simulink model "mmc_hb_switching"  (R2026a)
settings: Solver=ode3  StopTime=Tstop  FixedStep=Ts_elec
undefined symbols (not defined in the file): topology_id, Vdc, Vphase_cmd
libraries: fl_lib x23, nesl_utility x23, ee_lib x11
settings Model: Creator=zheng  LastModifiedBy=zheng

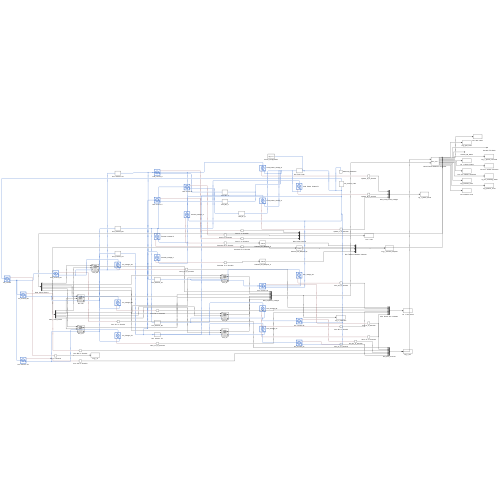
[thumbnail: Simulink's stored preview of the top-level diagram]
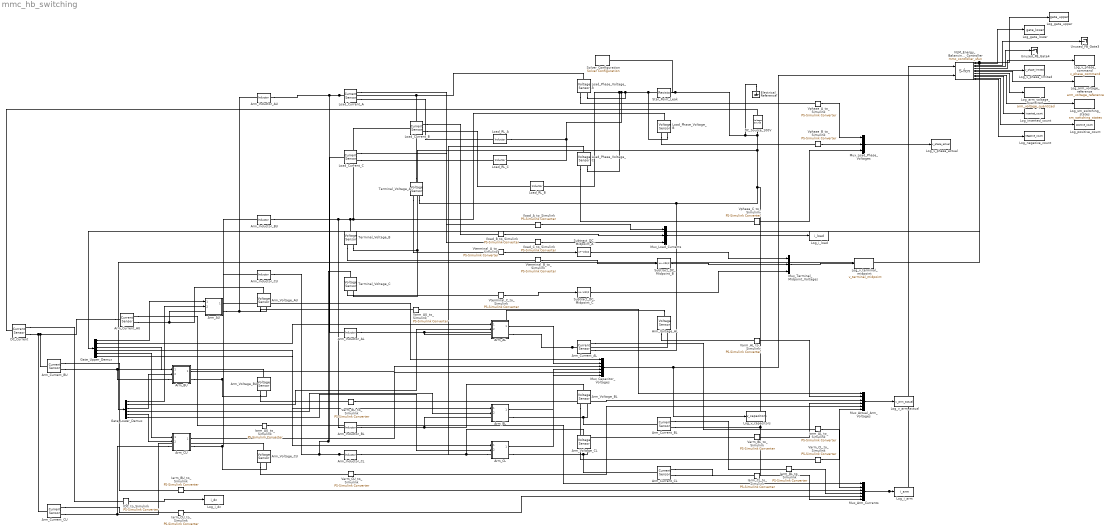
== system mmc_hb_switching ==
  Arm_AL : Subsystem  ReferencedSubsystem=mmc_hb_arm
  Arm_AU : Subsystem  ReferencedSubsystem=mmc_hb_arm
  Arm_BL : Subsystem  ReferencedSubsystem=mmc_hb_arm
  Arm_BU : Subsystem  ReferencedSubsystem=mmc_hb_arm
  Arm_CL : Subsystem  ReferencedSubsystem=mmc_hb_arm
  Arm_CU : Subsystem  ReferencedSubsystem=mmc_hb_arm
  Arm_Current_AL : fl_lib/Electrical/Electrical Sensors/Current Sensor
  Arm_Current_AU : fl_lib/Electrical/Electrical Sensors/Current Sensor
  Arm_Current_BL : fl_lib/Electrical/Electrical Sensors/Current Sensor
  Arm_Current_BU : fl_lib/Electrical/Electrical Sensors/Current Sensor
  Arm_Current_CL : fl_lib/Electrical/Electrical Sensors/Current Sensor
  Arm_Current_CU : fl_lib/Electrical/Electrical Sensors/Current Sensor
  Arm_Inductor_AL : ee_lib/Passive/Inductor  l=Larm H  enable_L_tol=ee.enum.toleranceApplication.none  L_tol=20  tol_distribution=ee.enum.toleranceDistribution.uniform  nSigma=4  r=Rarm Ohm  g=1e-9 1/Ohm  enable_operating_limits=ee.enum.enable.no  operating_limit_action=ee.enum.passive.reportOpLim.warn  max_working_current=1 A  power_rating=1 W  i_L_specify=off  i_L_priority=High  i_L=0 A  i_L_nominal_specify=off  i_L_nominal_value=1  i_L_nominal_unit=A
  Arm_Inductor_AU : ee_lib/Passive/Inductor  l=Larm H  enable_L_tol=ee.enum.toleranceApplication.none  L_tol=20  tol_distribution=ee.enum.toleranceDistribution.uniform  nSigma=4  r=Rarm Ohm  g=1e-9 1/Ohm  enable_operating_limits=ee.enum.enable.no  operating_limit_action=ee.enum.passive.reportOpLim.warn  max_working_current=1 A  power_rating=1 W  i_L_specify=off  i_L_priority=High  i_L=0 A  i_L_nominal_specify=off  i_L_nominal_value=1  i_L_nominal_unit=A
  Arm_Inductor_BL : ee_lib/Passive/Inductor  l=Larm H  enable_L_tol=ee.enum.toleranceApplication.none  L_tol=20  tol_distribution=ee.enum.toleranceDistribution.uniform  nSigma=4  r=Rarm Ohm  g=1e-9 1/Ohm  enable_operating_limits=ee.enum.enable.no  operating_limit_action=ee.enum.passive.reportOpLim.warn  max_working_current=1 A  power_rating=1 W  i_L_specify=off  i_L_priority=High  i_L=0 A  i_L_nominal_specify=off  i_L_nominal_value=1  i_L_nominal_unit=A
  Arm_Inductor_BU : ee_lib/Passive/Inductor  l=Larm H  enable_L_tol=ee.enum.toleranceApplication.none  L_tol=20  tol_distribution=ee.enum.toleranceDistribution.uniform  nSigma=4  r=Rarm Ohm  g=1e-9 1/Ohm  enable_operating_limits=ee.enum.enable.no  operating_limit_action=ee.enum.passive.reportOpLim.warn  max_working_current=1 A  power_rating=1 W  i_L_specify=off  i_L_priority=High  i_L=0 A  i_L_nominal_specify=off  i_L_nominal_value=1  i_L_nominal_unit=A
  Arm_Inductor_CL : ee_lib/Passive/Inductor  l=Larm H  enable_L_tol=ee.enum.toleranceApplication.none  L_tol=20  tol_distribution=ee.enum.toleranceDistribution.uniform  nSigma=4  r=Rarm Ohm  g=1e-9 1/Ohm  enable_operating_limits=ee.enum.enable.no  operating_limit_action=ee.enum.passive.reportOpLim.warn  max_working_current=1 A  power_rating=1 W  i_L_specify=off  i_L_priority=High  i_L=0 A  i_L_nominal_specify=off  i_L_nominal_value=1  i_L_nominal_unit=A
  Arm_Inductor_CU : ee_lib/Passive/Inductor  l=Larm H  enable_L_tol=ee.enum.toleranceApplication.none  L_tol=20  tol_distribution=ee.enum.toleranceDistribution.uniform  nSigma=4  r=Rarm Ohm  g=1e-9 1/Ohm  enable_operating_limits=ee.enum.enable.no  operating_limit_action=ee.enum.passive.reportOpLim.warn  max_working_current=1 A  power_rating=1 W  i_L_specify=off  i_L_priority=High  i_L=0 A  i_L_nominal_specify=off  i_L_nominal_value=1  i_L_nominal_unit=A
  Arm_Voltage_AL : fl_lib/Electrical/Electrical Sensors/Voltage Sensor
  Arm_Voltage_AU : fl_lib/Electrical/Electrical Sensors/Voltage Sensor
  Arm_Voltage_BL : fl_lib/Electrical/Electrical Sensors/Voltage Sensor
  Arm_Voltage_BU : fl_lib/Electrical/Electrical Sensors/Voltage Sensor
  Arm_Voltage_CL : fl_lib/Electrical/Electrical Sensors/Voltage Sensor
  Arm_Voltage_CU : fl_lib/Electrical/Electrical Sensors/Voltage Sensor
  DC_Current : fl_lib/Electrical/Electrical Sensors/Current Sensor
  DC_Source_100V : ee_lib/Sources/Voltage Source  dc_voltage=Vdc V  ac_voltage=0 V  ac_shift=0 rad  ac_frequency=60 Hz  noise_mode=ee.enum.sources.noise.Disabled  PSD=0 V^2/Hz  sample_time=1e-3 s  repeatability=ee.enum.sources.repeatability.NotRepeatable  user_seed=0  auto_seed=545404223  i_specify=off  i_priority=None  i=0 A  i_nominal_specify=off  i_nominal_value=1  i_nominal_unit=A  v_specify=off  v_priority=None  v=Vdc V  v_nominal_specify=off  v_nominal_value=1  v_nominal_unit=V
  Electrical_Reference : fl_lib/Electrical/Electrical Elements/Electrical Reference
  Gate_Lower_Demux : Demux  Outputs=[10 10 10 10 10 10]
  Gate_Upper_Demux : Demux  Outputs=[10 10 10 10 10 10]
  IDC_to_Simulink : nesl_utility/PS-Simulink Converter  PhysicalDomain=network_engine_domain  SubClassName=ps_output  LeftPortType=input  RightPortType=output  PseudoPeriodic=off  Frequencies=[]  VectorFormat=inherit  Unit=A  AffineConversion=off
  Iarm_AL_to_Simulink : nesl_utility/PS-Simulink Converter  PhysicalDomain=network_engine_domain  SubClassName=ps_output  LeftPortType=input  RightPortType=output  PseudoPeriodic=off  Frequencies=[]  VectorFormat=inherit  Unit=A  AffineConversion=off
  Iarm_AU_to_Simulink : nesl_utility/PS-Simulink Converter  PhysicalDomain=network_engine_domain  SubClassName=ps_output  LeftPortType=input  RightPortType=output  PseudoPeriodic=off  Frequencies=[]  VectorFormat=inherit  Unit=A  AffineConversion=off
  Iarm_BL_to_Simulink : nesl_utility/PS-Simulink Converter  PhysicalDomain=network_engine_domain  SubClassName=ps_output  LeftPortType=input  RightPortType=output  PseudoPeriodic=off  Frequencies=[]  VectorFormat=inherit  Unit=A  AffineConversion=off
  Iarm_BU_to_Simulink : nesl_utility/PS-Simulink Converter  PhysicalDomain=network_engine_domain  SubClassName=ps_output  LeftPortType=input  RightPortType=output  PseudoPeriodic=off  Frequencies=[]  VectorFormat=inherit  Unit=A  AffineConversion=off
  Iarm_CL_to_Simulink : nesl_utility/PS-Simulink Converter  PhysicalDomain=network_engine_domain  SubClassName=ps_output  LeftPortType=input  RightPortType=output  PseudoPeriodic=off  Frequencies=[]  VectorFormat=inherit  Unit=A  AffineConversion=off
  Iarm_CU_to_Simulink : nesl_utility/PS-Simulink Converter  PhysicalDomain=network_engine_domain  SubClassName=ps_output  LeftPortType=input  RightPortType=output  PseudoPeriodic=off  Frequencies=[]  VectorFormat=inherit  Unit=A  AffineConversion=off
  Iload_A_to_Simulink : nesl_utility/PS-Simulink Converter  PhysicalDomain=network_engine_domain  SubClassName=ps_output  LeftPortType=input  RightPortType=output  PseudoPeriodic=off  Frequencies=[]  VectorFormat=inherit  Unit=A  AffineConversion=off
  Iload_B_to_Simulink : nesl_utility/PS-Simulink Converter  PhysicalDomain=network_engine_domain  SubClassName=ps_output  LeftPortType=input  RightPortType=output  PseudoPeriodic=off  Frequencies=[]  VectorFormat=inherit  Unit=A  AffineConversion=off
  Iload_C_to_Simulink : nesl_utility/PS-Simulink Converter  PhysicalDomain=network_engine_domain  SubClassName=ps_output  LeftPortType=input  RightPortType=output  PseudoPeriodic=off  Frequencies=[]  VectorFormat=inherit  Unit=A  AffineConversion=off
  Load_Current_A : fl_lib/Electrical/Electrical Sensors/Current Sensor
  Load_Current_B : fl_lib/Electrical/Electrical Sensors/Current Sensor
  Load_Current_C : fl_lib/Electrical/Electrical Sensors/Current Sensor
  Load_Phase_Voltage_A : fl_lib/Electrical/Electrical Sensors/Voltage Sensor
  Load_Phase_Voltage_B : fl_lib/Electrical/Electrical Sensors/Voltage Sensor
  Load_Phase_Voltage_C : fl_lib/Electrical/Electrical Sensors/Voltage Sensor
  Load_RL_A : ee_lib/Passive/Inductor  l=Lload H  enable_L_tol=ee.enum.toleranceApplication.none  L_tol=20  tol_distribution=ee.enum.toleranceDistribution.uniform  nSigma=4  r=Rload Ohm  g=1e-9 1/Ohm  enable_operating_limits=ee.enum.enable.no  operating_limit_action=ee.enum.passive.reportOpLim.warn  max_working_current=1 A  power_rating=1 W  i_L_specify=off  i_L_priority=High  i_L=0 A  i_L_nominal_specify=off  i_L_nominal_value=1  i_L_nominal_unit=A
  Load_RL_B : ee_lib/Passive/Inductor  l=Lload H  enable_L_tol=ee.enum.toleranceApplication.none  L_tol=20  tol_distribution=ee.enum.toleranceDistribution.uniform  nSigma=4  r=Rload Ohm  g=1e-9 1/Ohm  enable_operating_limits=ee.enum.enable.no  operating_limit_action=ee.enum.passive.reportOpLim.warn  max_working_current=1 A  power_rating=1 W  i_L_specify=off  i_L_priority=High  i_L=0 A  i_L_nominal_specify=off  i_L_nominal_value=1  i_L_nominal_unit=A
  Load_RL_C : ee_lib/Passive/Inductor  l=Lload H  enable_L_tol=ee.enum.toleranceApplication.none  L_tol=20  tol_distribution=ee.enum.toleranceDistribution.uniform  nSigma=4  r=Rload Ohm  g=1e-9 1/Ohm  enable_operating_limits=ee.enum.enable.no  operating_limit_action=ee.enum.passive.reportOpLim.warn  max_working_current=1 A  power_rating=1 W  i_L_specify=off  i_L_priority=High  i_L=0 A  i_L_nominal_specify=off  i_L_nominal_value=1  i_L_nominal_unit=A
  Log_arm_voltage_quantized : ToWorkspace  VariableName=arm_voltage_quantized  SaveFormat=Timeseries  SampleTime=-1
  Log_arm_voltage_reference : ToWorkspace  VariableName=arm_voltage_reference  SaveFormat=Timeseries  SampleTime=-1
  Log_gate_lower : ToWorkspace  VariableName=gate_lower  SaveFormat=Timeseries  SampleTime=-1
  Log_gate_upper : ToWorkspace  VariableName=gate_upper  SaveFormat=Timeseries  SampleTime=-1
  Log_i_arm : ToWorkspace  VariableName=i_arm  SaveFormat=Timeseries  SampleTime=-1
  Log_i_dc : ToWorkspace  VariableName=i_dc  SaveFormat=Timeseries  SampleTime=-1
  Log_i_load : ToWorkspace  VariableName=i_load  SaveFormat=Timeseries  SampleTime=-1
  Log_inserted_count : ToWorkspace  VariableName=inserted_count  SaveFormat=Timeseries  SampleTime=-1
  Log_negative_count : ToWorkspace  VariableName=negative_count  SaveFormat=Timeseries  SampleTime=-1
  Log_positive_count : ToWorkspace  VariableName=positive_count  SaveFormat=Timeseries  SampleTime=-1
  Log_sm_switching_states : ToWorkspace  VariableName=sm_switching_states  SaveFormat=Timeseries  SampleTime=-1
  Log_v_arm_actual : ToWorkspace  VariableName=v_arm_actual  SaveFormat=Timeseries  SampleTime=-1
  Log_v_capacitors : ToWorkspace  VariableName=v_capacitors  SaveFormat=Timeseries  SampleTime=-1
  Log_v_phase_actual : ToWorkspace  VariableName=v_phase_actual  SaveFormat=Timeseries  SampleTime=-1
  Log_v_phase_command : ToWorkspace  VariableName=v_phase_command  SaveFormat=Timeseries  SampleTime=-1
  Log_v_phase_limited : ToWorkspace  VariableName=v_phase_limited  SaveFormat=Timeseries  SampleTime=-1
  Log_v_terminal_midpoint : ToWorkspace  VariableName=v_terminal_midpoint  SaveFormat=Timeseries  SampleTime=-1
  Mux_Actual_Arm_Voltages : Mux  Inputs=6
  Mux_Arm_Currents : Mux  Inputs=6
  Mux_Capacitor_Voltages : Mux  Inputs=6
  Mux_Load_Currents : Mux  Inputs=3
  Mux_Load_Phase_Voltages : Mux  Inputs=3
  Mux_Terminal_Midpoint_Voltages : Mux  Inputs=3
  NLM_Energy_Balancing_Controller : M-S-Function  FunctionName=mmc_controller_sfun  Parameters=topology_id,Vphase_cmd
  Solver_Configuration : nesl_utility/Solver Configuration  PhysicalDomain=network_engine_domain  SubClassName=solver  LeftPortType=input  RightPortType=generic  Tones=[]  Harmonics=[]  SimulateNoise=off  Profile=off  UseLocalSampling=off  EnableSwitchedLinearOptims=on  FrequencyDomain=off  UseCCode=off  RelTol=0.001  AbsTol=0.001  MinStep=1e-09  ToWorkspace=off  RevertToSquareIcSolve=off  NumHomotopyIterations=100  PhasorMode=off  PhasorModeNumHarmonics=1  ConsistencySolver=NEWTON_XTOL_AFTER_FTOL  CanonicalOrdering=CANONICAL  OptimizeIntermediates=OPTIMIZED  IndexReductionMethod=DerivativeReplacement  DoDC=off  ResidualTolerance=1e-09  ConsistencyTolSource=GLOBAL  ConsistencyAbsTol=0.001  ConsistencyRelTol=0.001  ConsistencyTolFactor=0.001  UseLocalSolver=on  LocalSolverChoice=NE_BACKWARD_EULER_ADVANCER  ResolveIndetEquations=on  FunctionEvalNumThread=1  LocalSolverSampleTime=Ts_elec  DoFixedCost=off  MaxNonlinIter=6  MaxModeIter=2  ComputeImpulses=off  ImpulseIterations=2  LinearAlgebra=auto  LinearAlgebraNumThread=0  EquationFormulation=NE_TIME_EF  DelaysMemoryBudget=1024  AutomaticFiltering=on  FilteringTimeConstant=0.001  PartitionStorageMethod=AS_NEEDED  PartitionMemoryBudget=1024  PartitionMethod=ROBUST  MultibodyUseLocalSolver=off  MultibodyLocalSolverChoice=ODE1  MultibodyLocalSolverSampleTime=0.001
  Star_Point_Leak : ee_lib/Passive/Resistor  R=1e9 Ohm  enable_R_tol=ee.enum.toleranceApplication.none  R_tol=5  tol_distribution=ee.enum.toleranceDistribution.uniform  nSigma=4  enable_operating_limits=ee.enum.enable.no  operating_limit_action=ee.enum.passive.reportOpLim.warn  power_rating=1 W  max_working_voltage=100 V  noise_mode=ee.enum.sources.noise.Disabled  Tdevice=25 degC  sample_time=1e-3 s  repeatability=ee.enum.ic.repeatability.notRepeatable  user_seed=0  auto_seed=3922919431  power_derating_T1=70 degC  power_derating_T2=155 degC  operating_temperature_range_vec=[-50, 150] degC  alpha=3.93e-3 1/K  Tmeas=25 degC  thermal_mass=100 J/K  temperature_specify=off  temperature_priority=High  temperature=298.15 K  temperature_nominal_specify=off  temperature_nominal_value=1  temperature_nominal_unit=K
  Subtract_DC_Midpoint_A : Bias  Bias=-Vdc/2
  Subtract_DC_Midpoint_B : Bias  Bias=-Vdc/2
  Subtract_DC_Midpoint_C : Bias  Bias=-Vdc/2
  Terminal_Voltage_A : fl_lib/Electrical/Electrical Sensors/Voltage Sensor
  Terminal_Voltage_B : fl_lib/Electrical/Electrical Sensors/Voltage Sensor
  Terminal_Voltage_C : fl_lib/Electrical/Electrical Sensors/Voltage Sensor
  Unused_FB_Gate3 : Terminator
  Unused_FB_Gate4 : Terminator
  Varm_AL_to_Simulink : nesl_utility/PS-Simulink Converter  PhysicalDomain=network_engine_domain  SubClassName=ps_output  LeftPortType=input  RightPortType=output  PseudoPeriodic=off  Frequencies=[]  VectorFormat=inherit  Unit=V  AffineConversion=off
  Varm_AU_to_Simulink : nesl_utility/PS-Simulink Converter  PhysicalDomain=network_engine_domain  SubClassName=ps_output  LeftPortType=input  RightPortType=output  PseudoPeriodic=off  Frequencies=[]  VectorFormat=inherit  Unit=V  AffineConversion=off
  Varm_BL_to_Simulink : nesl_utility/PS-Simulink Converter  PhysicalDomain=network_engine_domain  SubClassName=ps_output  LeftPortType=input  RightPortType=output  PseudoPeriodic=off  Frequencies=[]  VectorFormat=inherit  Unit=V  AffineConversion=off
  Varm_BU_to_Simulink : nesl_utility/PS-Simulink Converter  PhysicalDomain=network_engine_domain  SubClassName=ps_output  LeftPortType=input  RightPortType=output  PseudoPeriodic=off  Frequencies=[]  VectorFormat=inherit  Unit=V  AffineConversion=off
  Varm_CL_to_Simulink : nesl_utility/PS-Simulink Converter  PhysicalDomain=network_engine_domain  SubClassName=ps_output  LeftPortType=input  RightPortType=output  PseudoPeriodic=off  Frequencies=[]  VectorFormat=inherit  Unit=V  AffineConversion=off
  Varm_CU_to_Simulink : nesl_utility/PS-Simulink Converter  PhysicalDomain=network_engine_domain  SubClassName=ps_output  LeftPortType=input  RightPortType=output  PseudoPeriodic=off  Frequencies=[]  VectorFormat=inherit  Unit=V  AffineConversion=off
  Vphase_A_to_Simulink : nesl_utility/PS-Simulink Converter  PhysicalDomain=network_engine_domain  SubClassName=ps_output  LeftPortType=input  RightPortType=output  PseudoPeriodic=off  Frequencies=[]  VectorFormat=inherit  Unit=V  AffineConversion=off
  Vphase_B_to_Simulink : nesl_utility/PS-Simulink Converter  PhysicalDomain=network_engine_domain  SubClassName=ps_output  LeftPortType=input  RightPortType=output  PseudoPeriodic=off  Frequencies=[]  VectorFormat=inherit  Unit=V  AffineConversion=off
  Vphase_C_to_Simulink : nesl_utility/PS-Simulink Converter  PhysicalDomain=network_engine_domain  SubClassName=ps_output  LeftPortType=input  RightPortType=output  PseudoPeriodic=off  Frequencies=[]  VectorFormat=inherit  Unit=V  AffineConversion=off
  Vterminal_A_to_Simulink : nesl_utility/PS-Simulink Converter  PhysicalDomain=network_engine_domain  SubClassName=ps_output  LeftPortType=input  RightPortType=output  PseudoPeriodic=off  Frequencies=[]  VectorFormat=inherit  Unit=V  AffineConversion=off
  Vterminal_B_to_Simulink : nesl_utility/PS-Simulink Converter  PhysicalDomain=network_engine_domain  SubClassName=ps_output  LeftPortType=input  RightPortType=output  PseudoPeriodic=off  Frequencies=[]  VectorFormat=inherit  Unit=V  AffineConversion=off
  Vterminal_C_to_Simulink : nesl_utility/PS-Simulink Converter  PhysicalDomain=network_engine_domain  SubClassName=ps_output  LeftPortType=input  RightPortType=output  PseudoPeriodic=off  Frequencies=[]  VectorFormat=inherit  Unit=V  AffineConversion=off
  wires:
  Mux_Arm_Currents/1 -> Log_i_arm/1, NLM_Energy_Balancing_Controller/1
  Mux_Load_Phase_Voltages/1 -> Log_v_phase_actual/1
  Mux_Terminal_Midpoint_Voltages/1 -> Log_v_terminal_midpoint/1
  Mux_Load_Currents/1 -> Log_i_load/1
  Mux_Actual_Arm_Voltages/1 -> Log_v_arm_actual/1
  Mux_Capacitor_Voltages/1 -> NLM_Energy_Balancing_Controller/2, Log_v_capacitors/1
  IDC_to_Simulink/1 -> Log_i_dc/1
  Iarm_AU_to_Simulink/1 -> Mux_Arm_Currents/1
  Iarm_AL_to_Simulink/1 -> Mux_Arm_Currents/2
  Varm_AU_to_Simulink/1 -> Mux_Actual_Arm_Voltages/1
  Varm_AL_to_Simulink/1 -> Mux_Actual_Arm_Voltages/2
  Gate_Upper_Demux/2 -> Arm_AL/1
  Gate_Lower_Demux/2 -> Arm_AL/2
  Arm_AU/1 -> Mux_Capacitor_Voltages/1
  Arm_AL/1 -> Mux_Capacitor_Voltages/2
  Iload_A_to_Simulink/1 -> Mux_Load_Currents/1
  Vphase_A_to_Simulink/1 -> Mux_Load_Phase_Voltages/1
  Vterminal_A_to_Simulink/1 -> Subtract_DC_Midpoint_A/1
  Subtract_DC_Midpoint_A/1 -> Mux_Terminal_Midpoint_Voltages/1
  Iarm_BU_to_Simulink/1 -> Mux_Arm_Currents/3
  Iarm_BL_to_Simulink/1 -> Mux_Arm_Currents/4
  Varm_BU_to_Simulink/1 -> Mux_Actual_Arm_Voltages/3
  Varm_BL_to_Simulink/1 -> Mux_Actual_Arm_Voltages/4
  Gate_Upper_Demux/3 -> Arm_BU/1
  Gate_Lower_Demux/3 -> Arm_BU/2
  Gate_Upper_Demux/4 -> Arm_BL/1
  Gate_Lower_Demux/4 -> Arm_BL/2
  Arm_BU/1 -> Mux_Capacitor_Voltages/3
  Arm_BL/1 -> Mux_Capacitor_Voltages/4
  Iload_B_to_Simulink/1 -> Mux_Load_Currents/2
  Vphase_B_to_Simulink/1 -> Mux_Load_Phase_Voltages/2
  Vterminal_B_to_Simulink/1 -> Subtract_DC_Midpoint_B/1
  Subtract_DC_Midpoint_B/1 -> Mux_Terminal_Midpoint_Voltages/2
  Iarm_CU_to_Simulink/1 -> Mux_Arm_Currents/5
  Iarm_CL_to_Simulink/1 -> Mux_Arm_Currents/6
  Varm_CU_to_Simulink/1 -> Mux_Actual_Arm_Voltages/5
  Varm_CL_to_Simulink/1 -> Mux_Actual_Arm_Voltages/6
  Gate_Upper_Demux/5 -> Arm_CU/1
  Gate_Lower_Demux/5 -> Arm_CU/2
  Gate_Upper_Demux/6 -> Arm_CL/1
  Gate_Lower_Demux/6 -> Arm_CL/2
  Arm_CU/1 -> Mux_Capacitor_Voltages/5
  Arm_CL/1 -> Mux_Capacitor_Voltages/6
  Iload_C_to_Simulink/1 -> Mux_Load_Currents/3
  Vphase_C_to_Simulink/1 -> Mux_Load_Phase_Voltages/3
  Vterminal_C_to_Simulink/1 -> Subtract_DC_Midpoint_C/1
  Subtract_DC_Midpoint_C/1 -> Mux_Terminal_Midpoint_Voltages/3
  NLM_Energy_Balancing_Controller/1 -> Log_gate_upper/1, Gate_Upper_Demux/1
  NLM_Energy_Balancing_Controller/2 -> Log_gate_lower/1, Gate_Lower_Demux/1
  NLM_Energy_Balancing_Controller/3 -> Unused_FB_Gate3/1
  NLM_Energy_Balancing_Controller/4 -> Unused_FB_Gate4/1
  NLM_Energy_Balancing_Controller/5 -> Log_v_phase_command/1
  NLM_Energy_Balancing_Controller/6 -> Log_v_phase_limited/1
  NLM_Energy_Balancing_Controller/7 -> Log_arm_voltage_reference/1
  NLM_Energy_Balancing_Controller/8 -> Log_arm_voltage_quantized/1
  NLM_Energy_Balancing_Controller/9 -> Log_sm_switching_states/1
  NLM_Energy_Balancing_Controller/10 -> Log_inserted_count/1
  NLM_Energy_Balancing_Controller/11 -> Log_positive_count/1
  NLM_Energy_Balancing_Controller/12 -> Log_negative_count/1
  Gate_Upper_Demux/1 -> Arm_AU/1
  Gate_Lower_Demux/1 -> Arm_AU/2
  connections:
  DC_Source_100V/LConn1 -- DC_Current/LConn1
  DC_Current/RConn1 -- IDC_to_Simulink/LConn1
  Electrical_Reference/LConn1 -- Star_Point_Leak/RConn1 -- Solver_Configuration/RConn1 -- DC_Source_100V/RConn1 -- Terminal_Voltage_C/RConn2 -- Terminal_Voltage_B/RConn2 -- Arm_Current_CL/RConn2 -- Arm_Current_BL/RConn2 -- Arm_Current_AL/RConn2 -- Terminal_Voltage_A/RConn2
  Arm_Current_AU/LConn1 -- DC_Current/RConn2 -- Arm_Current_CU/LConn1 -- Arm_Current_BU/LConn1
  Arm_Current_AU/RConn2 -- Arm_AU/LConn1 -- Arm_Voltage_AU/LConn1
  Arm_AU/RConn1 -- Arm_Inductor_AU/LConn1 -- Arm_Voltage_AU/RConn2
  Terminal_Voltage_A/LConn1 -- Arm_Inductor_AU/RConn1 -- Arm_Inductor_AL/LConn1 -- Load_Current_A/LConn1 -- Load_Phase_Voltage_A/LConn1
  Arm_Voltage_AL/LConn1 -- Arm_Inductor_AL/RConn1 -- Arm_AL/LConn1
  Arm_AL/RConn1 -- Arm_Current_AL/LConn1 -- Arm_Voltage_AL/RConn2
  Load_Current_A/RConn2 -- Load_RL_A/LConn1
  Arm_Current_AU/RConn1 -- Iarm_AU_to_Simulink/LConn1
  Arm_Current_AL/RConn1 -- Iarm_AL_to_Simulink/LConn1
  Arm_Voltage_AU/RConn1 -- Varm_AU_to_Simulink/LConn1
  Arm_Voltage_AL/RConn1 -- Varm_AL_to_Simulink/LConn1
  Load_Current_A/RConn1 -- Iload_A_to_Simulink/LConn1
  Load_Phase_Voltage_A/RConn1 -- Vphase_A_to_Simulink/LConn1
  Terminal_Voltage_A/RConn1 -- Vterminal_A_to_Simulink/LConn1
  Arm_BU/LConn1 -- Arm_Current_BU/RConn2 -- Arm_Voltage_BU/LConn1
  Arm_BU/RConn1 -- Arm_Inductor_BU/LConn1 -- Arm_Voltage_BU/RConn2
  Arm_Inductor_BL/LConn1 -- Arm_Inductor_BU/RConn1 -- Load_Phase_Voltage_B/LConn1 -- Load_Current_B/LConn1 -- Terminal_Voltage_B/LConn1
  Arm_Inductor_BL/RConn1 -- Arm_BL/LConn1 -- Arm_Voltage_BL/LConn1
  Arm_BL/RConn1 -- Arm_Voltage_BL/RConn2 -- Arm_Current_BL/LConn1
  Load_Current_B/RConn2 -- Load_RL_B/LConn1
  Arm_Current_BU/RConn1 -- Iarm_BU_to_Simulink/LConn1
  Arm_Current_BL/RConn1 -- Iarm_BL_to_Simulink/LConn1
  Arm_Voltage_BU/RConn1 -- Varm_BU_to_Simulink/LConn1
  Arm_Voltage_BL/RConn1 -- Varm_BL_to_Simulink/LConn1
  Load_Current_B/RConn1 -- Iload_B_to_Simulink/LConn1
  Load_Phase_Voltage_B/RConn1 -- Vphase_B_to_Simulink/LConn1
  Terminal_Voltage_B/RConn1 -- Vterminal_B_to_Simulink/LConn1
  Arm_CU/LConn1 -- Arm_Current_CU/RConn2 -- Arm_Voltage_CU/LConn1
  Arm_CU/RConn1 -- Arm_Voltage_CU/RConn2 -- Arm_Inductor_CU/LConn1
  Arm_Inductor_CU/RConn1 -- Load_Phase_Voltage_C/LConn1 -- Arm_Inductor_CL/LConn1 -- Terminal_Voltage_C/LConn1 -- Load_Current_C/LConn1
  Arm_CL/LConn1 -- Arm_Inductor_CL/RConn1 -- Arm_Voltage_CL/LConn1
  Arm_CL/RConn1 -- Arm_Voltage_CL/RConn2 -- Arm_Current_CL/LConn1
  Load_Current_C/RConn2 -- Load_RL_C/LConn1
  Arm_Current_CU/RConn1 -- Iarm_CU_to_Simulink/LConn1
  Arm_Current_CL/RConn1 -- Iarm_CL_to_Simulink/LConn1
  Arm_Voltage_CU/RConn1 -- Varm_CU_to_Simulink/LConn1
  Arm_Voltage_CL/RConn1 -- Varm_CL_to_Simulink/LConn1
  Load_Current_C/RConn1 -- Iload_C_to_Simulink/LConn1
  Load_Phase_Voltage_C/RConn1 -- Vphase_C_to_Simulink/LConn1
  Terminal_Voltage_C/RConn1 -- Vterminal_C_to_Simulink/LConn1
  Load_RL_B/RConn1 -- Load_RL_A/RConn1 -- Load_RL_C/RConn1 -- Star_Point_Leak/LConn1 -- Load_Phase_Voltage_B/RConn2 -- Load_Phase_Voltage_A/RConn2 -- Load_Phase_Voltage_C/RConn2
